simulink model "l512_devel_pps_2016f"  (R2012b)
settings: Solver=ode45  StartTime=0.0  StopTime=15000  RelTol=1e-3
undefined symbols (not defined in the file): sfp
libraries: xbsIndex_r4 x7383, casper_library_misc x259, casper_library_delays x118, xps_library x12, simulink x1
(part 35 of 82)

== system l512_devel_pps_2016f/tenge/packetBuffer/b9 ==
  addressW : Inport
  addressR : Inport  Port=2
  data1 : Inport  Port=3
  data2 : Inport  Port=4
  data3 : Inport  Port=5
  data4 : Inport  Port=6
  AddSub : xbsIndex_r4/AddSub  mode=Addition  use_carryin=off  use_carryout=off  en=off  latency=1  precision=Full  arith_type=Unsigned  n_bits=10  bin_pt=0  quantization=Truncate  overflow=Wrap  dbl_ovrd=off  use_behavioral_HDL=off  hw_selection=Fabric  pipelined=off  block_type=addsub
  Constant : xbsIndex_r4/Constant  const=16382  gui_display_data_type=Fixed-point  arith_type=Unsigned  n_bits=14  bin_pt=0  preci_type=Single  exp_width=8  frac_width=24  explicit_period=off  period=1  equ=P=C  opselect=C  inp2=PCIN>>17  opr=+  inp1=P  carry=CIN  dbl_ovrd=off  block_type=constant
  Constant1 : xbsIndex_r4/Constant  const=436  gui_display_data_type=Fixed-point  arith_type=Unsigned  n_bits=9  bin_pt=0  preci_type=Single  exp_width=8  frac_width=24  explicit_period=on  period=1  equ=P=C  opselect=C  inp2=PCIN>>17  opr=+  inp1=P  carry=CIN  dbl_ovrd=off  block_type=constant
  Constant2 : xbsIndex_r4/Constant  const=869  gui_display_data_type=Fixed-point  arith_type=Unsigned  n_bits=10  bin_pt=0  preci_type=Single  exp_width=8  frac_width=24  explicit_period=on  period=1  equ=P=C  opselect=C  inp2=PCIN>>17  opr=+  inp1=P  carry=CIN  dbl_ovrd=off  block_type=constant
  Constant27 : xbsIndex_r4/Constant  const=870  gui_display_data_type=Fixed-point  arith_type=Unsigned  n_bits=10  bin_pt=0  preci_type=Single  exp_width=8  frac_width=24  explicit_period=on  period=1  equ=P=C  opselect=C  inp2=PCIN>>17  opr=+  inp1=P  carry=CIN  dbl_ovrd=off  block_type=constant
  Constant28 : xbsIndex_r4/Constant  const=218  gui_display_data_type=Fixed-point  arith_type=Unsigned  n_bits=9  bin_pt=0  preci_type=Single  exp_width=8  frac_width=24  explicit_period=on  period=1  equ=P=C  opselect=C  inp2=PCIN>>17  opr=+  inp1=P  carry=CIN  dbl_ovrd=off  block_type=constant
  Constant29 : xbsIndex_r4/Constant  const=654  gui_display_data_type=Fixed-point  arith_type=Unsigned  n_bits=10  bin_pt=0  preci_type=Single  exp_width=8  frac_width=24  explicit_period=on  period=1  equ=P=C  opselect=C  inp2=PCIN>>17  opr=+  inp1=P  carry=CIN  dbl_ovrd=off  block_type=constant
  Constant3 : xbsIndex_r4/Constant  const=871  gui_display_data_type=Fixed-point  arith_type=Unsigned  n_bits=10  bin_pt=0  preci_type=Single  exp_width=8  frac_width=24  explicit_period=on  period=1  equ=P=C  opselect=C  inp2=PCIN>>17  opr=+  inp1=P  carry=CIN  dbl_ovrd=off  block_type=constant
  Constant30 : xbsIndex_r4/Constant  const=109  gui_display_data_type=Fixed-point  arith_type=Unsigned  n_bits=9  bin_pt=0  preci_type=Single  exp_width=8  frac_width=24  explicit_period=on  period=1  equ=P=C  opselect=C  inp2=PCIN>>17  opr=+  inp1=P  carry=CIN  dbl_ovrd=off  block_type=constant
  Constant31 : xbsIndex_r4/Constant  const=327  gui_display_data_type=Fixed-point  arith_type=Unsigned  n_bits=10  bin_pt=0  preci_type=Single  exp_width=8  frac_width=24  explicit_period=on  period=1  equ=P=C  opselect=C  inp2=PCIN>>17  opr=+  inp1=P  carry=CIN  dbl_ovrd=off  block_type=constant
  Constant32 : xbsIndex_r4/Constant  const=545  gui_display_data_type=Fixed-point  arith_type=Unsigned  n_bits=10  bin_pt=0  preci_type=Single  exp_width=8  frac_width=24  explicit_period=on  period=1  equ=P=C  opselect=C  inp2=PCIN>>17  opr=+  inp1=P  carry=CIN  dbl_ovrd=off  block_type=constant
  Constant33 : xbsIndex_r4/Constant  const=763  gui_display_data_type=Fixed-point  arith_type=Unsigned  n_bits=10  bin_pt=0  preci_type=Single  exp_width=8  frac_width=24  explicit_period=on  period=1  equ=P=C  opselect=C  inp2=PCIN>>17  opr=+  inp1=P  carry=CIN  dbl_ovrd=off  block_type=constant
  Constant34 : xbsIndex_r4/Constant  const=108  gui_display_data_type=Fixed-point  arith_type=Unsigned  n_bits=9  bin_pt=0  preci_type=Single  exp_width=8  frac_width=24  explicit_period=on  period=1  equ=P=C  opselect=C  inp2=PCIN>>17  opr=+  inp1=P  carry=CIN  dbl_ovrd=off  block_type=constant
  Constant35 : xbsIndex_r4/Constant  const=0  gui_display_data_type=Fixed-point  arith_type=Unsigned  n_bits=9  bin_pt=0  preci_type=Single  exp_width=8  frac_width=24  explicit_period=on  period=1  equ=P=C  opselect=C  inp2=PCIN>>17  opr=+  inp1=P  carry=CIN  dbl_ovrd=off  block_type=constant
  Constant4 : xbsIndex_r4/Constant  const=870  gui_display_data_type=Fixed-point  arith_type=Unsigned  n_bits=10  bin_pt=0  preci_type=Single  exp_width=8  frac_width=24  explicit_period=off  period=1  equ=P=C  opselect=C  inp2=PCIN>>17  opr=+  inp1=P  carry=CIN  dbl_ovrd=off  block_type=constant
  Constant5 : xbsIndex_r4/Constant  const=870  gui_display_data_type=Fixed-point  arith_type=Unsigned  n_bits=10  bin_pt=0  preci_type=Single  exp_width=8  frac_width=24  explicit_period=off  period=1  equ=P=C  opselect=C  inp2=PCIN>>17  opr=+  inp1=P  carry=CIN  dbl_ovrd=off  block_type=constant
  Convert1 : xbsIndex_r4/Convert  gui_display_data_type=Fixed-point  arith_type=Unsigned  n_bits=10  bin_pt=0  float_type=Single  exp_bits=8  fraction_bits=24  quantization=Truncate  overflow=Wrap  en=off  latency=2  dbl_ovrd=off  pipeline=off  block_type=convert
      settings: block_version=11.4
  Convert2 : xbsIndex_r4/Convert  gui_display_data_type=Fixed-point  arith_type=Unsigned  n_bits=10  bin_pt=0  float_type=Single  exp_bits=8  fraction_bits=24  quantization=Truncate  overflow=Wrap  en=off  latency=2  dbl_ovrd=off  pipeline=off  block_type=convert
      settings: block_version=11.4
  Convert3 : xbsIndex_r4/Convert  gui_display_data_type=Boolean  arith_type=Boolean  n_bits=10  bin_pt=0  float_type=Single  exp_bits=8  fraction_bits=24  quantization=Truncate  overflow=Wrap  en=off  latency=1  dbl_ovrd=off  pipeline=off  block_type=convert
      settings: block_version=11.4
  Convert4 : xbsIndex_r4/Convert  gui_display_data_type=Boolean  arith_type=Boolean  n_bits=10  bin_pt=0  float_type=Single  exp_bits=8  fraction_bits=24  quantization=Truncate  overflow=Wrap  en=off  latency=0  dbl_ovrd=off  pipeline=off  block_type=convert
      settings: block_version=11.4
  Convert6 : xbsIndex_r4/Convert  gui_display_data_type=Boolean  arith_type=Boolean  n_bits=64  bin_pt=0  float_type=Single  exp_bits=8  fraction_bits=24  quantization=Truncate  overflow=Wrap  en=off  latency=0  dbl_ovrd=off  pipeline=off  block_type=convert
      settings: block_version=11.4
  Convert7 : xbsIndex_r4/Convert  gui_display_data_type=Boolean  arith_type=Boolean  n_bits=64  bin_pt=0  float_type=Single  exp_bits=8  fraction_bits=24  quantization=Truncate  overflow=Wrap  en=off  latency=0  dbl_ovrd=off  pipeline=off  block_type=convert
      settings: block_version=11.4
  Convert8 : xbsIndex_r4/Convert  gui_display_data_type=Boolean  arith_type=Boolean  n_bits=64  bin_pt=0  float_type=Single  exp_bits=8  fraction_bits=24  quantization=Truncate  overflow=Wrap  en=off  latency=0  dbl_ovrd=off  pipeline=off  block_type=convert
      settings: block_version=11.4
  Delay1 : xbsIndex_r4/Delay  rst=off  infoeditControl=Selection of Reset will increase slice count due to use of real FFs and instead of SRLs  en=off  latency=2  dbl_ovrd=off  reg_retiming=on  block_type=delay
  Delay2 : xbsIndex_r4/Delay  rst=off  infoeditControl=Selection of Reset will increase slice count due to use of real FFs and instead of SRLs  en=off  latency=3  dbl_ovrd=off  reg_retiming=on  block_type=delay
  Inverter2 : xbsIndex_r4/Inverter  en=off  latency=0  dbl_ovrd=off  block_type=inv
  Inverter3 : xbsIndex_r4/Inverter  en=off  latency=0  dbl_ovrd=off  block_type=inv
  Inverter4 : xbsIndex_r4/Inverter  en=off  latency=0  dbl_ovrd=off  block_type=inv
  Logical1 : xbsIndex_r4/Logical  logical_function=OR  inputs=2  en=off  latency=1  precision=Full  arith_type=Unsigned  n_bits=16  bin_pt=0  align_bp=on  dbl_ovrd=off  block_type=logical
      settings: block_version=11.4
  Logical14 : xbsIndex_r4/Logical  logical_function=AND  inputs=2  en=off  latency=1  precision=Full  arith_type=Unsigned  n_bits=16  bin_pt=0  align_bp=on  dbl_ovrd=off  block_type=logical
      settings: block_version=11.4
  Logical4 : xbsIndex_r4/Logical  logical_function=OR  inputs=2  en=off  latency=1  precision=Full  arith_type=Unsigned  n_bits=16  bin_pt=0  align_bp=on  dbl_ovrd=off  block_type=logical
      settings: block_version=11.4
  Mux : xbsIndex_r4/Mux  inputs=2  en=off  latency=0  precision=Full  arith_type=Unsigned  n_bits=16  bin_pt=14  quantization=Truncate  overflow=Wrap  dbl_ovrd=off  block_type=mux
  Mux1 : xbsIndex_r4/Mux  inputs=8  en=off  latency=2  precision=Full  arith_type="Signed  (2's comp)"  n_bits=8  bin_pt=2  quantization=Truncate  overflow=Wrap  dbl_ovrd=off  block_type=mux
      settings: xl_area=[0, 0, 0, 0, 0, 0, 0]
  Mux2 : xbsIndex_r4/Mux  inputs=4  en=off  latency=2  precision=Full  arith_type="Signed  (2's comp)"  n_bits=8  bin_pt=2  quantization=Truncate  overflow=Wrap  dbl_ovrd=off  block_type=mux
      settings: xl_area=[0, 0, 0, 0, 0, 0, 0]
  Mux3 : xbsIndex_r4/Mux  inputs=2  en=off  latency=0  precision=Full  arith_type=Unsigned  n_bits=16  bin_pt=14  quantization=Truncate  overflow=Wrap  dbl_ovrd=off  block_type=mux
  Mux4 : xbsIndex_r4/Mux  inputs=2  en=off  latency=0  precision=Full  arith_type=Unsigned  n_bits=16  bin_pt=14  quantization=Truncate  overflow=Wrap  dbl_ovrd=off  block_type=mux
  Relational{,2..3,28..29} (5 alike) : xbsIndex_r4/Relational  mode=a=b  en=off  latency=1  dbl_ovrd=off  block_type=relational
      Relational28 settings: xl_area=[0, 0, 0, 0, 0, 0, 0]  block_version=10.1.3
      Relational29 settings: xl_area=[0, 0, 0, 0, 0, 0, 0]  block_version=10.1.3
  Relational1 : xbsIndex_r4/Relational  mode=a<b  en=off  latency=1  dbl_ovrd=off  block_type=relational
      settings: xl_area=[0, 0, 0, 0, 0, 0, 0]  block_version=10.1.3
  Relational27 : xbsIndex_r4/Relational  mode=a=b  en=off  latency=0  dbl_ovrd=off  block_type=relational
      settings: xl_area=[0, 0, 0, 0, 0, 0, 0]  block_version=10.1.3
  Single Port RAM22 : xbsIndex_r4/Single Port RAM  depth=872  initVector=0  distributed_mem=Block RAM  write_mode=No Read On Write  rst=off  init_reg=0  en=off  latency=4  dbl_ovrd=off  optimize=Area  block_type=spram
  Single Port RAM23 : xbsIndex_r4/Single Port RAM  depth=872  initVector=0  distributed_mem=Block RAM  write_mode=No Read On Write  rst=off  init_reg=0  en=off  latency=4  dbl_ovrd=off  optimize=Area  block_type=spram
  buffer_cnt : xbsIndex_r4/Counter  cnt_type=Free Running  cnt_to=Inf  operation=Up  start_count=0  cnt_by_val=1  arith_type=Unsigned  n_bits=1  bin_pt=0  load_pin=off  rst=on  en=on  explicit_period=on  period=1  dbl_ovrd=off  use_behavioral_HDL=off  implementation=Fabric  block_type=counter
      settings: block_version=11.4
  edge_detect1 : Subsystem  AncestorBlock=casper_library_misc/edge_detect  mask(edge_detect){edge=Falling, polarity=Active High, x_in=[0 0.08 0.08 0.16 0.16 0.24 0.24 0.32 0.32 0.4], y_in=[1  1 -1 -1 -1 -1 -1 -1 -1 -1], x_out=[0.6 0.68 0.68 0.76 0.76 0.84 0.84 0.92 0.92 1], y_out=[-1 -1  1  1 -1 -1 -1 -1 -1 -1]}
      mask prompts: edge "Edge Type"; polarity "Output Polarity"; x_in "Input X Positions"; y_in "Input Y Positions"; x_out "Output X Positions"; y_out "Output Y Positions"
      mask help: Output is active for one-cycle after each edge of the specified type (i.e. rising, falling or both).
      mask init: same as l512_devel_pps_2016f/tenge/chSel/edge_detect2
      settings: AttributesFormatString=|
      | falling edges
      | active high
      mask Help: Output is active for one-cycle after each edge of the specified type (i.e. rising, falling, or both).  Latency is zero.
      mask TypeOptions edge: Rising | Falling | Both
      mask TypeOptions polarity: Active High | Active Low
      mask Display:
      | plot(x_in_num,0.5+y_in_num*0.2);
      | plot(x_out_num,0.5+y_out_num*0.2);
  edge_detect2 : Subsystem  AncestorBlock=casper_library_misc/edge_detect  mask(edge_detect){edge=Rising, polarity=Active High, x_in=[0 0.08 0.08 0.16 0.16 0.24 0.24 0.32 0.32 0.4], y_in=[-1 -1  1  1  1  1  1  1  1  1], x_out=[0.6 0.68 0.68 0.76 0.76 0.84 0.84 0.92 0.92 1], y_out=[-1 -1  1  1 -1 -1 -1 -1 -1 -1]}
      mask prompts: edge "Edge Type"; polarity "Output Polarity"; x_in "Input X Positions"; y_in "Input Y Positions"; x_out "Output X Positions"; y_out "Output Y Positions"
      mask help: Output is active for one-cycle after each edge of the specified type (i.e. rising, falling or both).
      mask init: same as l512_devel_pps_2016f/tenge/chSel/edge_detect2
      settings: AttributesFormatString=|
      | rising edges
      | active high
      mask Help: Output is active for one-cycle after each edge of the specified type (i.e. rising, falling, or both).  Latency is zero.
      mask TypeOptions edge: Rising | Falling | Both
      mask TypeOptions polarity: Active High | Active Low
      mask Display:
      | plot(x_in_num,0.5+y_in_num*0.2);
      | plot(x_out_num,0.5+y_out_num*0.2);
  edge_detect3 : Subsystem  AncestorBlock=casper_library_misc/edge_detect  mask(edge_detect){edge=Rising, polarity=Active High, x_in=[0 0.08 0.08 0.16 0.16 0.24 0.24 0.32 0.32 0.4], y_in=[-1 -1  1  1  1  1  1  1  1  1], x_out=[0.6 0.68 0.68 0.76 0.76 0.84 0.84 0.92 0.92 1], y_out=[-1 -1  1  1 -1 -1 -1 -1 -1 -1]}
      mask prompts: edge "Edge Type"; polarity "Output Polarity"; x_in "Input X Positions"; y_in "Input Y Positions"; x_out "Output X Positions"; y_out "Output Y Positions"
      mask help: Output is active for one-cycle after each edge of the specified type (i.e. rising, falling or both).
      mask init: same as l512_devel_pps_2016f/tenge/chSel/edge_detect2
      settings: AttributesFormatString=|
      | rising edges
      | active high
      mask Help: Output is active for one-cycle after each edge of the specified type (i.e. rising, falling, or both).  Latency is zero.
      mask TypeOptions edge: Rising | Falling | Both
      mask TypeOptions polarity: Active High | Active Low
      mask Display:
      | plot(x_in_num,0.5+y_in_num*0.2);
      | plot(x_out_num,0.5+y_out_num*0.2);
  edge_detect4 : Subsystem  AncestorBlock=casper_library_misc/edge_detect  mask(edge_detect){edge=Rising, polarity=Active High, x_in=[0 0.08 0.08 0.16 0.16 0.24 0.24 0.32 0.32 0.4], y_in=[-1 -1  1  1  1  1  1  1  1  1], x_out=[0.6 0.68 0.68 0.76 0.76 0.84 0.84 0.92 0.92 1], y_out=[-1 -1  1  1 -1 -1 -1 -1 -1 -1]}
      mask prompts: edge "Edge Type"; polarity "Output Polarity"; x_in "Input X Positions"; y_in "Input Y Positions"; x_out "Output X Positions"; y_out "Output Y Positions"
      mask help: Output is active for one-cycle after each edge of the specified type (i.e. rising, falling or both).
      mask init: same as l512_devel_pps_2016f/tenge/chSel/edge_detect2
      settings: AttributesFormatString=|
      | rising edges
      | active high
      mask Help: Output is active for one-cycle after each edge of the specified type (i.e. rising, falling, or both).  Latency is zero.
      mask TypeOptions edge: Rising | Falling | Both
      mask TypeOptions polarity: Active High | Active Low
      mask Display:
      | plot(x_in_num,0.5+y_in_num*0.2);
      | plot(x_out_num,0.5+y_out_num*0.2);
  posedge : casper_library_misc/posedge  Tag=Rising Edge Detector
  posedge1 : casper_library_misc/posedge  Tag=Rising Edge Detector
  system_counter1 : xbsIndex_r4/Counter  cnt_type=Count Limited  cnt_to=7  operation=Up  start_count=0  cnt_by_val=1  arith_type=Unsigned  n_bits=3  bin_pt=0  load_pin=off  rst=on  en=on  explicit_period=on  period=1  dbl_ovrd=off  use_behavioral_HDL=off  implementation=Fabric  block_type=counter
      settings: block_version=11.4
  system_counter2 : xbsIndex_r4/Counter  cnt_type=Free Running  cnt_to=7  operation=Up  start_count=0  cnt_by_val=1  arith_type=Unsigned  n_bits=2  bin_pt=0  load_pin=off  rst=on  en=on  explicit_period=on  period=1  dbl_ovrd=off  use_behavioral_HDL=off  implementation=Fabric  block_type=counter
      settings: block_version=11.4
  system_counter3 : xbsIndex_r4/Counter  cnt_type=Count Limited  cnt_to=108  operation=Up  start_count=0  cnt_by_val=1  arith_type=Unsigned  n_bits=7  bin_pt=0  load_pin=off  rst=on  en=on  explicit_period=on  period=1  dbl_ovrd=off  use_behavioral_HDL=off  implementation=Fabric  block_type=counter
      settings: block_version=11.4
  system_counter4 : xbsIndex_r4/Counter  cnt_type=Count Limited  cnt_to=871  operation=Up  start_count=0  cnt_by_val=1  arith_type=Unsigned  n_bits=10  bin_pt=0  load_pin=off  rst=on  en=on  explicit_period=on  period=1  dbl_ovrd=off  use_behavioral_HDL=off  implementation=Fabric  block_type=counter
      settings: block_version=11.4
  system_counter5 : xbsIndex_r4/Counter  cnt_type=Free Running  cnt_to=871  operation=Up  start_count=0  cnt_by_val=1  arith_type=Unsigned  n_bits=32  bin_pt=0  load_pin=off  rst=on  en=on  explicit_period=on  period=1  dbl_ovrd=off  use_behavioral_HDL=off  implementation=Fabric  block_type=counter
      settings: block_version=11.4
  system_counter6 : xbsIndex_r4/Counter  cnt_type=Free Running  cnt_to=16384  operation=Up  start_count=0  cnt_by_val=1  arith_type=Unsigned  n_bits=14  bin_pt=0  load_pin=off  rst=on  en=off  explicit_period=on  period=1  dbl_ovrd=off  use_behavioral_HDL=off  implementation=Fabric  block_type=counter
      settings: block_version=11.4
  system_counter7 : xbsIndex_r4/Counter  cnt_type=Free Running  cnt_to=16384  operation=Up  start_count=0  cnt_by_val=1  arith_type=Unsigned  n_bits=1  bin_pt=0  load_pin=off  rst=on  en=on  explicit_period=on  period=1  dbl_ovrd=off  use_behavioral_HDL=off  implementation=Fabric  block_type=counter
      settings: block_version=11.4
  system_counter8 : xbsIndex_r4/Counter  cnt_type=Free Running  cnt_to=16384  operation=Up  start_count=0  cnt_by_val=1  arith_type=Unsigned  n_bits=1  bin_pt=0  load_pin=off  rst=on  en=on  explicit_period=on  period=1  dbl_ovrd=off  use_behavioral_HDL=off  implementation=Fabric  block_type=counter
      settings: block_version=11.4
  system_counter9 : xbsIndex_r4/Counter  cnt_type=Free Running  cnt_to=16384  operation=Up  start_count=0  cnt_by_val=1  arith_type=Unsigned  n_bits=1  bin_pt=0  load_pin=off  rst=on  en=on  explicit_period=on  period=1  dbl_ovrd=off  use_behavioral_HDL=off  implementation=Fabric  block_type=counter
      settings: block_version=11.4
  eof_10g : Outport
  valid_10g : Outport  Port=2
  dataOut : Outport  Port=3
  wires:
  Mux/1 -> dataOut/1
  Inverter4/1 -> Single Port RAM22/3
  Inverter3/1 -> Single Port RAM23/3
  Convert8/1 -> Inverter4/1
  Convert6/1 -> Inverter3/1
  system_counter9/1 -> Convert8/1  "wea"
  posedge1/1 -> system_counter9/2
  [cnt_rst] -> system_counter9/1
  Relational3/1 -> posedge1/1
  Constant5/1 -> Relational3/1
  posedge/1 -> system_counter8/2
  [cnt_rst] -> system_counter8/1
  system_counter8/1 -> Convert6/1  "web"
  Relational2/1 -> posedge/1
  Constant4/1 -> Relational2/1
  Mux3/1 -> Single Port RAM23/1, Relational2/2
  Convert7/1 -> Inverter2/1, Mux3/1
  Inverter2/1 -> Mux4/1
  system_counter7/1 -> Convert7/1, Mux/1
  Mux4/1 -> Single Port RAM22/1, Relational3/2
  Convert1/1 -> Mux4/3, Mux3/3
  Relational/1 -> system_counter7/2
  Constant/1 -> Relational/1
  system_counter6/1 -> Relational/2  "sel"
  [cnt_rst] -> system_counter7/1
  [sync_rnd] -> system_counter6/1
  Single Port RAM23/1 -> Mux/3
  Single Port RAM22/1 -> Mux/2
  buffer_cnt/1 -> Convert4/1
  Logical4/1 -> buffer_cnt/2
  AddSub/1 -> Relational28/2, Convert2/1
  Relational28/1 -> edge_detect3/1(in)
  edge_detect4/1(out) -> Logical4/2, Convert3/1
  Relational29/1 -> edge_detect4/1(in)
  Constant27/1 -> Relational28/1
  [offset_incW] -> Mux1/1
  Constant35/1 -> Mux1/2
  Constant28/1 -> Mux1/3
  Constant1/1 -> Mux1/4
  Constant29/1 -> Mux1/5
  Constant30/1 -> Mux1/6
  Constant31/1 -> Mux1/7
  Constant32/1 -> Mux1/8
  Constant33/1 -> Mux1/9
  system_counter3/1 -> Relational27/2, Delay1/1
  Mux1/1 -> AddSub/2
  Constant34/1 -> Relational27/1
  Relational27/1 -> edge_detect2/1(in)
  [cnt_rst] -> system_counter3/1
  system_counter4/1 -> Relational29/2, Convert1/1
  [cnt_rst] -> system_counter4/1
  addressW/1 -> system_counter3/2
  addressR/1 -> system_counter4/2
  edge_detect2/1(out) -> system_counter1/2, system_counter2/2
  system_counter1/1 -> [offset_incW]
  [cnt_rst] -> system_counter1/1, system_counter2/1
  Convert2/1 -> Mux4/2, Mux3/2
  Delay1/1 -> AddSub/1
  Convert3/1 -> eof_10g/1  "eof"
  Convert4/1 -> edge_detect1/1(in), Logical14/2, system_counter5/2  "valid"
  system_counter2/1 -> Delay2/1, [data_inc]  "data_inc"
  data1/1 -> Mux2/2
  data2/1 -> Mux2/3
  data3/1 -> Mux2/4
  data4/1 -> Mux2/5
  Mux2/1 -> Single Port RAM23/2, Single Port RAM22/2  "data"
  Constant2/1 -> Relational29/1
  Constant3/1 -> Relational1/2
  system_counter5/1 -> Relational1/1
  [cnt_rst] -> Logical1/1
  edge_detect1/1(out) -> Logical1/2
  Logical1/1 -> system_counter5/1
  Relational1/1 -> Logical14/1
  Logical14/1 -> valid_10g/1
  Delay2/1 -> Mux2/1
  [cnt_rst] -> buffer_cnt/1
  edge_detect3/1(out) -> Logical4/1

== system l512_devel_pps_2016f/tenge/packetBuffer/delay_valid1 ==
  in : Inport
  Gateway Out{2..3,55..56} (4 alike) : xbsIndex_r4/Gateway Out  inherit_from_input=off  hdl_port=on  timing_constraint=None  locs_specified=off  LOCs={}  UseAsDAC=off  DACChannel='1'  block_type=gatewayout
      settings: infoedit="Gateway out block.  Converts Xilinx fixed point inputs into ouputs of type Simulink integer, double, or fixed point.<P><P>Hardware notes:  In hardware these blocks become top level output ports or are discarded, depending on how they are configured."  xl_area=[0, 0, 0, 0, 0, 0, 0]  block_version=9.2.01
  Register : xbsIndex_r4/Register  init=0  rst=on  en=on  dbl_ovrd=off  block_type=register
      settings: xl_area=[0, 0, 0, 0, 0, 0, 0]  block_version=9.2.01
  Scope2 : Scope  NumInputPorts=4
      settings: YMin=0~0~0~-1  YMax=1~1~1~1  SaveName=ScopeData16
  negedge : casper_library_misc/negedge  Tag=Rising Edge Detector
  posedge : casper_library_misc/posedge  Tag=Rising Edge Detector
  sync_delay : casper_library_delays/sync_delay  DelayLen=delay-1
  sync_delay1 : casper_library_delays/sync_delay  DelayLen=delay-1
  out : Outport
  wires:
  sync_delay1/1 -> Register/2, Gateway Out2/1
  Gateway Out56/1 -> Scope2/2
  Register/1 -> out/1, Gateway Out3/1
  Gateway Out55/1 -> Scope2/1
  Gateway Out3/1 -> Scope2/4
  sync_delay/1 -> Register/1, Register/3, Gateway Out56/1
  in/1 -> negedge/1, posedge/1, Gateway Out55/1
  negedge/1 -> sync_delay1/1
  Gateway Out2/1 -> Scope2/3
  posedge/1 -> sync_delay/1

== system l512_devel_pps_2016f/tenge/packetBuffer/delay_valid10 ==
  in : Inport
  Gateway Out{2..3,55..56} (4 alike) : xbsIndex_r4/Gateway Out  inherit_from_input=off  hdl_port=on  timing_constraint=None  locs_specified=off  LOCs={}  UseAsDAC=off  DACChannel='1'  block_type=gatewayout
      settings: infoedit="Gateway out block.  Converts Xilinx fixed point inputs into ouputs of type Simulink integer, double, or fixed point.<P><P>Hardware notes:  In hardware these blocks become top level output ports or are discarded, depending on how they are configured."  xl_area=[0, 0, 0, 0, 0, 0, 0]  block_version=9.2.01
  Register : xbsIndex_r4/Register  init=0  rst=on  en=on  dbl_ovrd=off  block_type=register
      settings: xl_area=[0, 0, 0, 0, 0, 0, 0]  block_version=9.2.01
  Scope2 : Scope  NumInputPorts=4
      settings: YMin=0~0~0~-1  YMax=1~1~1~1  SaveName=ScopeData16
  negedge : casper_library_misc/negedge  Tag=Rising Edge Detector
  posedge : casper_library_misc/posedge  Tag=Rising Edge Detector
  sync_delay : casper_library_delays/sync_delay  DelayLen=delay-1
  sync_delay1 : casper_library_delays/sync_delay  DelayLen=delay-1
  out : Outport
  wires:
  posedge/1 -> sync_delay/1
  Gateway Out2/1 -> Scope2/3
  negedge/1 -> sync_delay1/1
  in/1 -> Gateway Out55/1, posedge/1, negedge/1
  sync_delay/1 -> Gateway Out56/1, Register/3, Register/1
  Gateway Out3/1 -> Scope2/4
  Gateway Out55/1 -> Scope2/1
  Register/1 -> Gateway Out3/1, out/1
  Gateway Out56/1 -> Scope2/2
  sync_delay1/1 -> Gateway Out2/1, Register/2

== system l512_devel_pps_2016f/tenge/packetBuffer/delay_valid11 ==
  in : Inport
  Gateway Out{2..3,55..56} (4 alike) : xbsIndex_r4/Gateway Out  inherit_from_input=off  hdl_port=on  timing_constraint=None  locs_specified=off  LOCs={}  UseAsDAC=off  DACChannel='1'  block_type=gatewayout
      settings: infoedit="Gateway out block.  Converts Xilinx fixed point inputs into ouputs of type Simulink integer, double, or fixed point.<P><P>Hardware notes:  In hardware these blocks become top level output ports or are discarded, depending on how they are configured."  xl_area=[0, 0, 0, 0, 0, 0, 0]  block_version=9.2.01
  Register : xbsIndex_r4/Register  init=0  rst=on  en=on  dbl_ovrd=off  block_type=register
      settings: xl_area=[0, 0, 0, 0, 0, 0, 0]  block_version=9.2.01
  Scope2 : Scope  NumInputPorts=4
      settings: YMin=0~0~0~-1  YMax=1~1~1~1  SaveName=ScopeData16
  negedge : casper_library_misc/negedge  Tag=Rising Edge Detector
  posedge : casper_library_misc/posedge  Tag=Rising Edge Detector
  sync_delay : casper_library_delays/sync_delay  DelayLen=delay-1
  sync_delay1 : casper_library_delays/sync_delay  DelayLen=delay-1
  out : Outport
  wires:
  posedge/1 -> sync_delay/1
  Gateway Out2/1 -> Scope2/3
  negedge/1 -> sync_delay1/1
  in/1 -> Gateway Out55/1, posedge/1, negedge/1
  sync_delay/1 -> Gateway Out56/1, Register/3, Register/1
  Gateway Out3/1 -> Scope2/4
  Gateway Out55/1 -> Scope2/1
  Register/1 -> Gateway Out3/1, out/1
  Gateway Out56/1 -> Scope2/2
  sync_delay1/1 -> Gateway Out2/1, Register/2

== system l512_devel_pps_2016f/tenge/packetBuffer/delay_valid12 ==
  in : Inport
  Gateway Out{2..3,55..56} (4 alike) : xbsIndex_r4/Gateway Out  inherit_from_input=off  hdl_port=on  timing_constraint=None  locs_specified=off  LOCs={}  UseAsDAC=off  DACChannel='1'  block_type=gatewayout
      settings: infoedit="Gateway out block.  Converts Xilinx fixed point inputs into ouputs of type Simulink integer, double, or fixed point.<P><P>Hardware notes:  In hardware these blocks become top level output ports or are discarded, depending on how they are configured."  xl_area=[0, 0, 0, 0, 0, 0, 0]  block_version=9.2.01
  Register : xbsIndex_r4/Register  init=0  rst=on  en=on  dbl_ovrd=off  block_type=register
      settings: xl_area=[0, 0, 0, 0, 0, 0, 0]  block_version=9.2.01
  Scope2 : Scope  NumInputPorts=4
      settings: YMin=0~0~0~-1  YMax=1~1~1~1  SaveName=ScopeData16
  negedge : casper_library_misc/negedge  Tag=Rising Edge Detector
  posedge : casper_library_misc/posedge  Tag=Rising Edge Detector
  sync_delay : casper_library_delays/sync_delay  DelayLen=delay-1
  sync_delay1 : casper_library_delays/sync_delay  DelayLen=delay-1
  out : Outport
  wires:
  posedge/1 -> sync_delay/1
  Gateway Out2/1 -> Scope2/3
  negedge/1 -> sync_delay1/1
  in/1 -> Gateway Out55/1, posedge/1, negedge/1
  sync_delay/1 -> Gateway Out56/1, Register/3, Register/1
  Gateway Out3/1 -> Scope2/4
  Gateway Out55/1 -> Scope2/1
  Register/1 -> Gateway Out3/1, out/1
  Gateway Out56/1 -> Scope2/2
  sync_delay1/1 -> Gateway Out2/1, Register/2

== system l512_devel_pps_2016f/tenge/packetBuffer/delay_valid13 ==
  in : Inport
  Gateway Out{2..3,55..56} (4 alike) : xbsIndex_r4/Gateway Out  inherit_from_input=off  hdl_port=on  timing_constraint=None  locs_specified=off  LOCs={}  UseAsDAC=off  DACChannel='1'  block_type=gatewayout
      settings: infoedit="Gateway out block.  Converts Xilinx fixed point inputs into ouputs of type Simulink integer, double, or fixed point.<P><P>Hardware notes:  In hardware these blocks become top level output ports or are discarded, depending on how they are configured."  xl_area=[0, 0, 0, 0, 0, 0, 0]  block_version=9.2.01
  Register : xbsIndex_r4/Register  init=0  rst=on  en=on  dbl_ovrd=off  block_type=register
      settings: xl_area=[0, 0, 0, 0, 0, 0, 0]  block_version=9.2.01
  Scope2 : Scope  NumInputPorts=4
      settings: YMin=0~0~0~-1  YMax=1~1~1~1  SaveName=ScopeData16
  negedge : casper_library_misc/negedge  Tag=Rising Edge Detector
  posedge : casper_library_misc/posedge  Tag=Rising Edge Detector
  sync_delay : casper_library_delays/sync_delay  DelayLen=delay-1
  sync_delay1 : casper_library_delays/sync_delay  DelayLen=delay-1
  out : Outport
  wires:
  posedge/1 -> sync_delay/1
  Gateway Out2/1 -> Scope2/3
  negedge/1 -> sync_delay1/1
  in/1 -> Gateway Out55/1, posedge/1, negedge/1
  sync_delay/1 -> Gateway Out56/1, Register/3, Register/1
  Gateway Out3/1 -> Scope2/4
  Gateway Out55/1 -> Scope2/1
  Register/1 -> Gateway Out3/1, out/1
  Gateway Out56/1 -> Scope2/2
  sync_delay1/1 -> Gateway Out2/1, Register/2

== system l512_devel_pps_2016f/tenge/packetBuffer/delay_valid14 ==
  in : Inport
  Gateway Out{2..3,55..56} (4 alike) : xbsIndex_r4/Gateway Out  inherit_from_input=off  hdl_port=on  timing_constraint=None  locs_specified=off  LOCs={}  UseAsDAC=off  DACChannel='1'  block_type=gatewayout
      settings: infoedit="Gateway out block.  Converts Xilinx fixed point inputs into ouputs of type Simulink integer, double, or fixed point.<P><P>Hardware notes:  In hardware these blocks become top level output ports or are discarded, depending on how they are configured."  xl_area=[0, 0, 0, 0, 0, 0, 0]  block_version=9.2.01
  Register : xbsIndex_r4/Register  init=0  rst=on  en=on  dbl_ovrd=off  block_type=register
      settings: xl_area=[0, 0, 0, 0, 0, 0, 0]  block_version=9.2.01
  Scope2 : Scope  NumInputPorts=4
      settings: YMin=0~0~0~-1  YMax=1~1~1~1  SaveName=ScopeData16
  negedge : casper_library_misc/negedge  Tag=Rising Edge Detector
  posedge : casper_library_misc/posedge  Tag=Rising Edge Detector
  sync_delay : casper_library_delays/sync_delay  DelayLen=delay-1
  sync_delay1 : casper_library_delays/sync_delay  DelayLen=delay-1
  out : Outport
  wires:
  posedge/1 -> sync_delay/1
  Gateway Out2/1 -> Scope2/3
  negedge/1 -> sync_delay1/1
  in/1 -> Gateway Out55/1, posedge/1, negedge/1
  sync_delay/1 -> Gateway Out56/1, Register/3, Register/1
  Gateway Out3/1 -> Scope2/4
  Gateway Out55/1 -> Scope2/1
  Register/1 -> Gateway Out3/1, out/1
  Gateway Out56/1 -> Scope2/2
  sync_delay1/1 -> Gateway Out2/1, Register/2

== system l512_devel_pps_2016f/tenge/packetBuffer/delay_valid15 ==
  in : Inport
  Gateway Out{2..3,55..56} (4 alike) : xbsIndex_r4/Gateway Out  inherit_from_input=off  hdl_port=on  timing_constraint=None  locs_specified=off  LOCs={}  UseAsDAC=off  DACChannel='1'  block_type=gatewayout
      settings: infoedit="Gateway out block.  Converts Xilinx fixed point inputs into ouputs of type Simulink integer, double, or fixed point.<P><P>Hardware notes:  In hardware these blocks become top level output ports or are discarded, depending on how they are configured."  xl_area=[0, 0, 0, 0, 0, 0, 0]  block_version=9.2.01
  Register : xbsIndex_r4/Register  init=0  rst=on  en=on  dbl_ovrd=off  block_type=register
      settings: xl_area=[0, 0, 0, 0, 0, 0, 0]  block_version=9.2.01
  Scope2 : Scope  NumInputPorts=4
      settings: YMin=0~0~0~-1  YMax=1~1~1~1  SaveName=ScopeData16
  negedge : casper_library_misc/negedge  Tag=Rising Edge Detector
  posedge : casper_library_misc/posedge  Tag=Rising Edge Detector
  sync_delay : casper_library_delays/sync_delay  DelayLen=delay-1
  sync_delay1 : casper_library_delays/sync_delay  DelayLen=delay-1
  out : Outport
  wires:
  posedge/1 -> sync_delay/1
  Gateway Out2/1 -> Scope2/3
  negedge/1 -> sync_delay1/1
  in/1 -> Gateway Out55/1, posedge/1, negedge/1
  sync_delay/1 -> Gateway Out56/1, Register/3, Register/1
  Gateway Out3/1 -> Scope2/4
  Gateway Out55/1 -> Scope2/1
  Register/1 -> Gateway Out3/1, out/1
  Gateway Out56/1 -> Scope2/2
  sync_delay1/1 -> Gateway Out2/1, Register/2

== system l512_devel_pps_2016f/tenge/packetBuffer/delay_valid16 ==
  in : Inport
  Gateway Out{2..3,55..56} (4 alike) : xbsIndex_r4/Gateway Out  inherit_from_input=off  hdl_port=on  timing_constraint=None  locs_specified=off  LOCs={}  UseAsDAC=off  DACChannel='1'  block_type=gatewayout
      settings: infoedit="Gateway out block.  Converts Xilinx fixed point inputs into ouputs of type Simulink integer, double, or fixed point.<P><P>Hardware notes:  In hardware these blocks become top level output ports or are discarded, depending on how they are configured."  xl_area=[0, 0, 0, 0, 0, 0, 0]  block_version=9.2.01
  Register : xbsIndex_r4/Register  init=0  rst=on  en=on  dbl_ovrd=off  block_type=register
      settings: xl_area=[0, 0, 0, 0, 0, 0, 0]  block_version=9.2.01
  Scope2 : Scope  NumInputPorts=4
      settings: YMin=0~0~0~-1  YMax=1~1~1~1  SaveName=ScopeData16
  negedge : casper_library_misc/negedge  Tag=Rising Edge Detector
  posedge : casper_library_misc/posedge  Tag=Rising Edge Detector
  sync_delay : casper_library_delays/sync_delay  DelayLen=delay-1
  sync_delay1 : casper_library_delays/sync_delay  DelayLen=delay-1
  out : Outport
  wires:
  sync_delay1/1 -> Register/2, Gateway Out2/1
  Gateway Out56/1 -> Scope2/2
  Register/1 -> out/1, Gateway Out3/1
  Gateway Out55/1 -> Scope2/1
  Gateway Out3/1 -> Scope2/4
  sync_delay/1 -> Register/1, Register/3, Gateway Out56/1
  in/1 -> negedge/1, posedge/1, Gateway Out55/1
  negedge/1 -> sync_delay1/1
  Gateway Out2/1 -> Scope2/3
  posedge/1 -> sync_delay/1

== system l512_devel_pps_2016f/tenge/packetBuffer/delay_valid17 ==
  in : Inport
  Gateway Out{2..3,55..56} (4 alike) : xbsIndex_r4/Gateway Out  inherit_from_input=off  hdl_port=on  timing_constraint=None  locs_specified=off  LOCs={}  UseAsDAC=off  DACChannel='1'  block_type=gatewayout
      settings: infoedit="Gateway out block.  Converts Xilinx fixed point inputs into ouputs of type Simulink integer, double, or fixed point.<P><P>Hardware notes:  In hardware these blocks become top level output ports or are discarded, depending on how they are configured."  xl_area=[0, 0, 0, 0, 0, 0, 0]  block_version=9.2.01
  Register : xbsIndex_r4/Register  init=0  rst=on  en=on  dbl_ovrd=off  block_type=register
      settings: xl_area=[0, 0, 0, 0, 0, 0, 0]  block_version=9.2.01
  Scope2 : Scope  NumInputPorts=4
      settings: YMin=0~0~0~-1  YMax=1~1~1~1  SaveName=ScopeData16
  negedge : casper_library_misc/negedge  Tag=Rising Edge Detector
  posedge : casper_library_misc/posedge  Tag=Rising Edge Detector
  sync_delay : casper_library_delays/sync_delay  DelayLen=delay-1
  sync_delay1 : casper_library_delays/sync_delay  DelayLen=delay-1
  out : Outport
  wires:
  sync_delay1/1 -> Register/2, Gateway Out2/1
  Gateway Out56/1 -> Scope2/2
  Register/1 -> out/1, Gateway Out3/1
  Gateway Out55/1 -> Scope2/1
  Gateway Out3/1 -> Scope2/4
  sync_delay/1 -> Register/1, Register/3, Gateway Out56/1
  in/1 -> negedge/1, posedge/1, Gateway Out55/1
  negedge/1 -> sync_delay1/1
  Gateway Out2/1 -> Scope2/3
  posedge/1 -> sync_delay/1

== system l512_devel_pps_2016f/tenge/packetBuffer/delay_valid18 ==
  in : Inport
  Gateway Out{2..3,55..56} (4 alike) : xbsIndex_r4/Gateway Out  inherit_from_input=off  hdl_port=on  timing_constraint=None  locs_specified=off  LOCs={}  UseAsDAC=off  DACChannel='1'  block_type=gatewayout
      settings: infoedit="Gateway out block.  Converts Xilinx fixed point inputs into ouputs of type Simulink integer, double, or fixed point.<P><P>Hardware notes:  In hardware these blocks become top level output ports or are discarded, depending on how they are configured."  xl_area=[0, 0, 0, 0, 0, 0, 0]  block_version=9.2.01
  Register : xbsIndex_r4/Register  init=0  rst=on  en=on  dbl_ovrd=off  block_type=register
      settings: xl_area=[0, 0, 0, 0, 0, 0, 0]  block_version=9.2.01
  Scope2 : Scope  NumInputPorts=4
      settings: YMin=0~0~0~-1  YMax=1~1~1~1  SaveName=ScopeData16
  negedge : casper_library_misc/negedge  Tag=Rising Edge Detector
  posedge : casper_library_misc/posedge  Tag=Rising Edge Detector
  sync_delay : casper_library_delays/sync_delay  DelayLen=delay-1
  sync_delay1 : casper_library_delays/sync_delay  DelayLen=delay-1
  out : Outport
  wires:
  sync_delay1/1 -> Register/2, Gateway Out2/1
  Gateway Out56/1 -> Scope2/2
  Register/1 -> out/1, Gateway Out3/1
  Gateway Out55/1 -> Scope2/1
  Gateway Out3/1 -> Scope2/4
  sync_delay/1 -> Register/1, Register/3, Gateway Out56/1
  in/1 -> negedge/1, posedge/1, Gateway Out55/1
  negedge/1 -> sync_delay1/1
  Gateway Out2/1 -> Scope2/3
  posedge/1 -> sync_delay/1

== system l512_devel_pps_2016f/tenge/packetBuffer/delay_valid19 ==
  in : Inport
  Gateway Out{2..3,55..56} (4 alike) : xbsIndex_r4/Gateway Out  inherit_from_input=off  hdl_port=on  timing_constraint=None  locs_specified=off  LOCs={}  UseAsDAC=off  DACChannel='1'  block_type=gatewayout
      settings: infoedit="Gateway out block.  Converts Xilinx fixed point inputs into ouputs of type Simulink integer, double, or fixed point.<P><P>Hardware notes:  In hardware these blocks become top level output ports or are discarded, depending on how they are configured."  xl_area=[0, 0, 0, 0, 0, 0, 0]  block_version=9.2.01
  Register : xbsIndex_r4/Register  init=0  rst=on  en=on  dbl_ovrd=off  block_type=register
      settings: xl_area=[0, 0, 0, 0, 0, 0, 0]  block_version=9.2.01
  Scope2 : Scope  NumInputPorts=4
      settings: YMin=0~0~0~-1  YMax=1~1~1~1  SaveName=ScopeData16
  negedge : casper_library_misc/negedge  Tag=Rising Edge Detector
  posedge : casper_library_misc/posedge  Tag=Rising Edge Detector
  sync_delay : casper_library_delays/sync_delay  DelayLen=delay-1
  sync_delay1 : casper_library_delays/sync_delay  DelayLen=delay-1
  out : Outport
  wires:
  sync_delay1/1 -> Register/2, Gateway Out2/1
  Gateway Out56/1 -> Scope2/2
  Register/1 -> out/1, Gateway Out3/1
  Gateway Out55/1 -> Scope2/1
  Gateway Out3/1 -> Scope2/4
  sync_delay/1 -> Register/1, Register/3, Gateway Out56/1
  in/1 -> negedge/1, posedge/1, Gateway Out55/1
  negedge/1 -> sync_delay1/1
  Gateway Out2/1 -> Scope2/3
  posedge/1 -> sync_delay/1

== system l512_devel_pps_2016f/tenge/packetBuffer/delay_valid2 ==
  in : Inport
  Gateway Out{2..3,55..56} (4 alike) : xbsIndex_r4/Gateway Out  inherit_from_input=off  hdl_port=on  timing_constraint=None  locs_specified=off  LOCs={}  UseAsDAC=off  DACChannel='1'  block_type=gatewayout
      settings: infoedit="Gateway out block.  Converts Xilinx fixed point inputs into ouputs of type Simulink integer, double, or fixed point.<P><P>Hardware notes:  In hardware these blocks become top level output ports or are discarded, depending on how they are configured."  xl_area=[0, 0, 0, 0, 0, 0, 0]  block_version=9.2.01
  Register : xbsIndex_r4/Register  init=0  rst=on  en=on  dbl_ovrd=off  block_type=register
      settings: xl_area=[0, 0, 0, 0, 0, 0, 0]  block_version=9.2.01
  Scope2 : Scope  NumInputPorts=4
      settings: YMin=0~0~0~-1  YMax=1~1~1~1  SaveName=ScopeData16
  negedge : casper_library_misc/negedge  Tag=Rising Edge Detector
  posedge : casper_library_misc/posedge  Tag=Rising Edge Detector
  sync_delay : casper_library_delays/sync_delay  DelayLen=delay-1
  sync_delay1 : casper_library_delays/sync_delay  DelayLen=delay-1
  out : Outport
  wires:
  sync_delay1/1 -> Register/2, Gateway Out2/1
  Gateway Out56/1 -> Scope2/2
  Register/1 -> out/1, Gateway Out3/1
  Gateway Out55/1 -> Scope2/1
  Gateway Out3/1 -> Scope2/4
  sync_delay/1 -> Register/1, Register/3, Gateway Out56/1
  in/1 -> negedge/1, posedge/1, Gateway Out55/1
  negedge/1 -> sync_delay1/1
  Gateway Out2/1 -> Scope2/3
  posedge/1 -> sync_delay/1

== system l512_devel_pps_2016f/tenge/packetBuffer/delay_valid20 ==
  in : Inport
  Gateway Out{2..3,55..56} (4 alike) : xbsIndex_r4/Gateway Out  inherit_from_input=off  hdl_port=on  timing_constraint=None  locs_specified=off  LOCs={}  UseAsDAC=off  DACChannel='1'  block_type=gatewayout
      settings: infoedit="Gateway out block.  Converts Xilinx fixed point inputs into ouputs of type Simulink integer, double, or fixed point.<P><P>Hardware notes:  In hardware these blocks become top level output ports or are discarded, depending on how they are configured."  xl_area=[0, 0, 0, 0, 0, 0, 0]  block_version=9.2.01
  Register : xbsIndex_r4/Register  init=0  rst=on  en=on  dbl_ovrd=off  block_type=register
      settings: xl_area=[0, 0, 0, 0, 0, 0, 0]  block_version=9.2.01
  Scope2 : Scope  NumInputPorts=4
      settings: YMin=0~0~0~-1  YMax=1~1~1~1  SaveName=ScopeData16
  negedge : casper_library_misc/negedge  Tag=Rising Edge Detector
  posedge : casper_library_misc/posedge  Tag=Rising Edge Detector
  sync_delay : casper_library_delays/sync_delay  DelayLen=delay-1
  sync_delay1 : casper_library_delays/sync_delay  DelayLen=delay-1
  out : Outport
  wires:
  sync_delay1/1 -> Register/2, Gateway Out2/1
  Gateway Out56/1 -> Scope2/2
  Register/1 -> out/1, Gateway Out3/1
  Gateway Out55/1 -> Scope2/1
  Gateway Out3/1 -> Scope2/4
  sync_delay/1 -> Register/1, Register/3, Gateway Out56/1
  in/1 -> negedge/1, posedge/1, Gateway Out55/1
  negedge/1 -> sync_delay1/1
  Gateway Out2/1 -> Scope2/3
  posedge/1 -> sync_delay/1

== system l512_devel_pps_2016f/tenge/packetBuffer/delay_valid21 ==
  in : Inport
  Gateway Out{2..3,55..56} (4 alike) : xbsIndex_r4/Gateway Out  inherit_from_input=off  hdl_port=on  timing_constraint=None  locs_specified=off  LOCs={}  UseAsDAC=off  DACChannel='1'  block_type=gatewayout
      settings: infoedit="Gateway out block.  Converts Xilinx fixed point inputs into ouputs of type Simulink integer, double, or fixed point.<P><P>Hardware notes:  In hardware these blocks become top level output ports or are discarded, depending on how they are configured."  xl_area=[0, 0, 0, 0, 0, 0, 0]  block_version=9.2.01
  Register : xbsIndex_r4/Register  init=0  rst=on  en=on  dbl_ovrd=off  block_type=register
      settings: xl_area=[0, 0, 0, 0, 0, 0, 0]  block_version=9.2.01
  Scope2 : Scope  NumInputPorts=4
      settings: YMin=0~0~0~-1  YMax=1~1~1~1  SaveName=ScopeData16
  negedge : casper_library_misc/negedge  Tag=Rising Edge Detector
  posedge : casper_library_misc/posedge  Tag=Rising Edge Detector
  sync_delay : casper_library_delays/sync_delay  DelayLen=delay-1
  sync_delay1 : casper_library_delays/sync_delay  DelayLen=delay-1
  out : Outport
  wires:
  sync_delay1/1 -> Register/2, Gateway Out2/1
  Gateway Out56/1 -> Scope2/2
  Register/1 -> out/1, Gateway Out3/1
  Gateway Out55/1 -> Scope2/1
  Gateway Out3/1 -> Scope2/4
  sync_delay/1 -> Register/1, Register/3, Gateway Out56/1
  in/1 -> negedge/1, posedge/1, Gateway Out55/1
  negedge/1 -> sync_delay1/1
  Gateway Out2/1 -> Scope2/3
  posedge/1 -> sync_delay/1

== system l512_devel_pps_2016f/tenge/packetBuffer/delay_valid22 ==
  in : Inport
  Gateway Out{2..3,55..56} (4 alike) : xbsIndex_r4/Gateway Out  inherit_from_input=off  hdl_port=on  timing_constraint=None  locs_specified=off  LOCs={}  UseAsDAC=off  DACChannel='1'  block_type=gatewayout
      settings: infoedit="Gateway out block.  Converts Xilinx fixed point inputs into ouputs of type Simulink integer, double, or fixed point.<P><P>Hardware notes:  In hardware these blocks become top level output ports or are discarded, depending on how they are configured."  xl_area=[0, 0, 0, 0, 0, 0, 0]  block_version=9.2.01
  Register : xbsIndex_r4/Register  init=0  rst=on  en=on  dbl_ovrd=off  block_type=register
      settings: xl_area=[0, 0, 0, 0, 0, 0, 0]  block_version=9.2.01
  Scope2 : Scope  NumInputPorts=4
      settings: YMin=0~0~0~-1  YMax=1~1~1~1  SaveName=ScopeData16
  negedge : casper_library_misc/negedge  Tag=Rising Edge Detector
  posedge : casper_library_misc/posedge  Tag=Rising Edge Detector
  sync_delay : casper_library_delays/sync_delay  DelayLen=delay-1
  sync_delay1 : casper_library_delays/sync_delay  DelayLen=delay-1
  out : Outport
  wires:
  sync_delay1/1 -> Register/2, Gateway Out2/1
  Gateway Out56/1 -> Scope2/2
  Register/1 -> out/1, Gateway Out3/1
  Gateway Out55/1 -> Scope2/1
  Gateway Out3/1 -> Scope2/4
  sync_delay/1 -> Register/1, Register/3, Gateway Out56/1
  in/1 -> negedge/1, posedge/1, Gateway Out55/1
  negedge/1 -> sync_delay1/1
  Gateway Out2/1 -> Scope2/3
  posedge/1 -> sync_delay/1

== system l512_devel_pps_2016f/tenge/packetBuffer/delay_valid23 ==
  in : Inport
  Gateway Out{2..3,55..56} (4 alike) : xbsIndex_r4/Gateway Out  inherit_from_input=off  hdl_port=on  timing_constraint=None  locs_specified=off  LOCs={}  UseAsDAC=off  DACChannel='1'  block_type=gatewayout
      settings: infoedit="Gateway out block.  Converts Xilinx fixed point inputs into ouputs of type Simulink integer, double, or fixed point.<P><P>Hardware notes:  In hardware these blocks become top level output ports or are discarded, depending on how they are configured."  xl_area=[0, 0, 0, 0, 0, 0, 0]  block_version=9.2.01
  Register : xbsIndex_r4/Register  init=0  rst=on  en=on  dbl_ovrd=off  block_type=register
      settings: xl_area=[0, 0, 0, 0, 0, 0, 0]  block_version=9.2.01
  Scope2 : Scope  NumInputPorts=4
      settings: YMin=0~0~0~-1  YMax=1~1~1~1  SaveName=ScopeData16
  negedge : casper_library_misc/negedge  Tag=Rising Edge Detector
  posedge : casper_library_misc/posedge  Tag=Rising Edge Detector
  sync_delay : casper_library_delays/sync_delay  DelayLen=delay-1
  sync_delay1 : casper_library_delays/sync_delay  DelayLen=delay-1
  out : Outport
  wires:
  sync_delay1/1 -> Register/2, Gateway Out2/1
  Gateway Out56/1 -> Scope2/2
  Register/1 -> out/1, Gateway Out3/1
  Gateway Out55/1 -> Scope2/1
  Gateway Out3/1 -> Scope2/4
  sync_delay/1 -> Register/1, Register/3, Gateway Out56/1
  in/1 -> negedge/1, posedge/1, Gateway Out55/1
  negedge/1 -> sync_delay1/1
  Gateway Out2/1 -> Scope2/3
  posedge/1 -> sync_delay/1

== system l512_devel_pps_2016f/tenge/packetBuffer/delay_valid24 ==
  in : Inport
  Gateway Out{2..3,55..56} (4 alike) : xbsIndex_r4/Gateway Out  inherit_from_input=off  hdl_port=on  timing_constraint=None  locs_specified=off  LOCs={}  UseAsDAC=off  DACChannel='1'  block_type=gatewayout
      settings: infoedit="Gateway out block.  Converts Xilinx fixed point inputs into ouputs of type Simulink integer, double, or fixed point.<P><P>Hardware notes:  In hardware these blocks become top level output ports or are discarded, depending on how they are configured."  xl_area=[0, 0, 0, 0, 0, 0, 0]  block_version=9.2.01
  Register : xbsIndex_r4/Register  init=0  rst=on  en=on  dbl_ovrd=off  block_type=register
      settings: xl_area=[0, 0, 0, 0, 0, 0, 0]  block_version=9.2.01
  Scope2 : Scope  NumInputPorts=4
      settings: YMin=0~0~0~-1  YMax=1~1~1~1  SaveName=ScopeData16
  negedge : casper_library_misc/negedge  Tag=Rising Edge Detector
  posedge : casper_library_misc/posedge  Tag=Rising Edge Detector
  sync_delay : casper_library_delays/sync_delay  DelayLen=delay-1
  sync_delay1 : casper_library_delays/sync_delay  DelayLen=delay-1
  out : Outport
  wires:
  sync_delay1/1 -> Register/2, Gateway Out2/1
  Gateway Out56/1 -> Scope2/2
  Register/1 -> out/1, Gateway Out3/1
  Gateway Out55/1 -> Scope2/1
  Gateway Out3/1 -> Scope2/4
  sync_delay/1 -> Register/1, Register/3, Gateway Out56/1
  in/1 -> negedge/1, posedge/1, Gateway Out55/1
  negedge/1 -> sync_delay1/1
  Gateway Out2/1 -> Scope2/3
  posedge/1 -> sync_delay/1

== system l512_devel_pps_2016f/tenge/packetBuffer/delay_valid25 ==
  in : Inport
  Gateway Out{2..3,55..56} (4 alike) : xbsIndex_r4/Gateway Out  inherit_from_input=off  hdl_port=on  timing_constraint=None  locs_specified=off  LOCs={}  UseAsDAC=off  DACChannel='1'  block_type=gatewayout
      settings: infoedit="Gateway out block.  Converts Xilinx fixed point inputs into ouputs of type Simulink integer, double, or fixed point.<P><P>Hardware notes:  In hardware these blocks become top level output ports or are discarded, depending on how they are configured."  xl_area=[0, 0, 0, 0, 0, 0, 0]  block_version=9.2.01
  Register : xbsIndex_r4/Register  init=0  rst=on  en=on  dbl_ovrd=off  block_type=register
      settings: xl_area=[0, 0, 0, 0, 0, 0, 0]  block_version=9.2.01
  Scope2 : Scope  NumInputPorts=4
      settings: YMin=0~0~0~-1  YMax=1~1~1~1  SaveName=ScopeData16
  negedge : casper_library_misc/negedge  Tag=Rising Edge Detector
  posedge : casper_library_misc/posedge  Tag=Rising Edge Detector
  sync_delay : casper_library_delays/sync_delay  DelayLen=delay-1
  sync_delay1 : casper_library_delays/sync_delay  DelayLen=delay-1
  out : Outport
  wires:
  sync_delay1/1 -> Register/2, Gateway Out2/1
  Gateway Out56/1 -> Scope2/2
  Register/1 -> out/1, Gateway Out3/1
  Gateway Out55/1 -> Scope2/1
  Gateway Out3/1 -> Scope2/4
  sync_delay/1 -> Register/1, Register/3, Gateway Out56/1
  in/1 -> negedge/1, posedge/1, Gateway Out55/1
  negedge/1 -> sync_delay1/1
  Gateway Out2/1 -> Scope2/3
  posedge/1 -> sync_delay/1
